simulink model "plotting_sim"  (R2014b)
settings: Solver=ode45  StartTime=0.0  StopTime=15  FixedStep=ts  RelTol=1e-3
values from neighbouring files (symbols this model uses):
  A = eval(As)    [plotting_script.m]
  B = eval(Bs)    [plotting_script.m]
  Cc = eye(5,6)    [plotting_script.m]
  Kr = (-inv(Cs*inv(Aa-Bb*K)*Bb))    [plotting_script.m]
undefined symbols (not defined in the file or in its folder): K, sigbuilder_block
settings Model: CovSFcnEnable=on  Creator=Jaby  LastModifiedBy=danielpihlquist
settings OptimizationCC: UseDivisionForNetSlopeComputation=off  SimCompilerOptimization=off
settings DebuggingCC: SolverPrmCheckMsg=none  FrameProcessingCompatibilityMsg=error
settings RTWCC: RTWCompilerOptimization=off

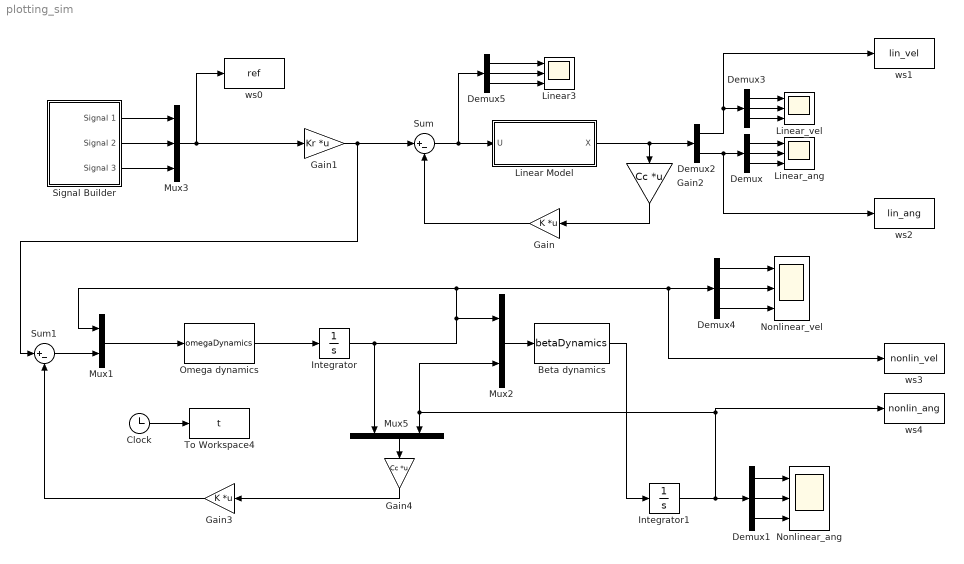
== system plotting_sim ==
  Beta dynamics : MATLABFcn  MATLABFcn=betaDynamics  Output1D=off
  Clock : Clock
  Demux{,1,3..5} (5 alike) : Demux  Outputs=3
  Demux2 : Demux  Outputs=2
  Gain : Gain  Gain=K  Multiplication=Matrix(K*u)
  Gain1 : Gain  Gain=Kr  Multiplication=Matrix(K*u)
  Gain2 : Gain  Gain=Cc  Multiplication=Matrix(K*u)
  Gain3 : Gain  Gain=K  Multiplication=Matrix(K*u)
  Gain4 : Gain  Gain=Cc  Multiplication=Matrix(K*u)
  Integrator : Integrator  InitialCondition=[0 0 0]'
  Integrator1 : Integrator  InitialCondition=[0 0 0]'
  "Linear Model " : Subsystem
  Linear3 : Scope  NumInputPorts=3
      settings: TimeRange=20  YMin=0.00274~-3.07e-14~8.3e-31  YMax=0.00278~-3.025e-14~8.43e-31  SaveName=ScopeData4
  Linear_ang : Scope  NumInputPorts=3
      settings: TimeRange=20  YMin=0.00274~-3.07e-14~8.3e-31  YMax=0.00278~-3.025e-14~8.43e-31
  Linear_vel : Scope  NumInputPorts=3
      settings: TimeRange=20  YMin=-0.5~-0.5~0  YMax=2.5~2.5~0.7000000000000001  SaveName=ScopeData2
  Mux1 : Mux  Inputs=2
  Mux2 : Mux  Inputs=2
  Mux3 : Mux  Inputs=3
  Mux5 : Mux  Inputs=2
  "Nonlinear_ang " : Scope  NumInputPorts=3
      settings: YMin=-5~-5~-5  YMax=5~5~5
  Nonlinear_vel : Scope  NumInputPorts=3
      settings: YMin=-5~-5~-5  YMax=5~5~5  SaveName=ScopeData3
  Omega dynamics : MATLABFcn  MATLABFcn=omegaDynamics  Output1D=off
  Signal Builder : Subsystem  Tag=STV Subsys  LoadFcn=sigbuilder_block('load');  StartFcn=sigbuilder_block('start');  StopFcn=sigbuilder_block('stop');  ClipboardFcn=sigbuilder_block('clipboard');  mask(Sigbuilder block){}
      mask help: Simulink:masks:SigbuilderBlock_MD
      mask init:
      | if ~strcmp(get_param(bdroot(gcbh),'SimulationStatus'),'stopped') tuvar = sigbuilder_block('maskInit'); end
      settings: CopyFcn=sigbuilder_block('copy');  DeleteFcn=sigbuilder_block('delete');  ModelCloseFcn=sigbuilder_block('modelClose');  PreSaveFcn=sigbuilder_block('preSave');  PauseFcn=sigbuilder_block('pause');  ContinueFcn=sigbuilder_block('continue');  NameChangeFcn=sigbuilder_block('namechange');  OpenFcn=sigbuilder_block('open',[437.6 199.2 550.4 400 ]);  CloseFcn=sigbuilder_block('close');
      mask Display: plot(0, 0, 100, 100,[2, 2, 32, 32, 2], [68, 8, 8, 68, 68],[32, 2], [38, 38], [32, 19, 2],[53, 60, 44], [32, 17, 17, 2],[16, 16, 31, 31]);txt = getActiveGroup(gcbh);text(2, 100, txt,'verticalAlignment', 'top');
  Sum : Sum  Inputs=|+-
  Sum1 : Sum  Inputs=|+-
  To Workspace4 : ToWorkspace  VariableName=t  SampleTime=-1
  ws0 : ToWorkspace  VariableName=ref  SampleTime=-1
  ws1 : ToWorkspace  VariableName=lin_vel  SampleTime=-1
  ws2 : ToWorkspace  VariableName=lin_ang  SampleTime=-1
  ws3 : ToWorkspace  VariableName=nonlin_vel  SampleTime=-1
  ws4 : ToWorkspace  VariableName=nonlin_ang  SampleTime=-1
  wires:
  Demux/1 -> Linear_ang/1
  Demux/2 -> Linear_ang/2
  Demux/3 -> Linear_ang/3
  Integrator/1 -> Demux4/1, ws3/1, Mux1/1, Mux2/1, Mux5/1
  Mux1/1 -> Omega dynamics/1
  Omega dynamics/1 -> Integrator/1
  Beta dynamics/1 -> Integrator1/1
  Demux1/2 -> "Nonlinear_ang "/2
  Demux1/3 -> "Nonlinear_ang "/3
  Demux1/1 -> "Nonlinear_ang "/1
  Gain/1 -> Sum/2
  Demux2/2 -> Demux/1, ws2/1
  Signal Builder/2(Signal 2) -> Mux3/2
  Signal Builder/1(Signal 1) -> Mux3/1
  Demux3/1 -> Linear_vel/1
  Demux3/2 -> Linear_vel/2
  Demux3/3 -> Linear_vel/3
  Signal Builder/3(Signal 3) -> Mux3/3
  "Linear Model "/1(X) -> Demux2/1, Gain2/1
  Gain1/1 -> Sum1/1, Sum/1
  Demux5/1 -> Linear3/1
  Demux5/2 -> Linear3/2
  Demux5/3 -> Linear3/3
  Sum/1 -> Demux5/1, "Linear Model "/1(U)
  Gain2/1 -> Gain/1
  Gain4/1 -> Gain3/1
  Gain3/1 -> Sum1/2
  Sum1/1 -> Mux1/2
  Mux5/1 -> Gain4/1
  Demux4/2 -> Nonlinear_vel/2
  Mux2/1 -> Beta dynamics/1
  Demux4/3 -> Nonlinear_vel/3
  Demux4/1 -> Nonlinear_vel/1
  Mux3/1 -> Gain1/1, ws0/1
  Demux2/1 -> Demux3/1, ws1/1
  Integrator1/1 -> Demux1/1, ws4/1, Mux5/2, Mux2/2
  Clock/1 -> To Workspace4/1

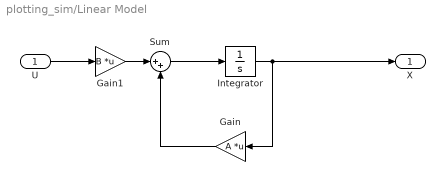
== system plotting_sim/Linear Model  ==
  U : Inport
  Gain : Gain  Gain=A  Multiplication=Matrix(K*u)
  Gain1 : Gain  Gain=B  Multiplication=Matrix(K*u)
  Integrator : Integrator
  Sum : Sum  Inputs=|++
  X : Outport
  wires:
  Integrator/1 -> X/1, Gain/1
  U/1 -> Gain1/1
  Gain1/1 -> Sum/1
  Sum/1 -> Integrator/1
  Gain/1 -> Sum/2

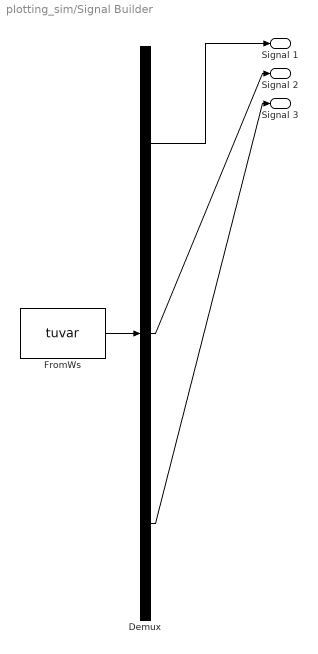
== system plotting_sim/Signal Builder ==
  Demux : Demux  Tag=STV Demux  Outputs=3
  FromWs : FromWorkspace  Tag=STV FromWs  VariableName=tuvar  SampleTime=0
      SigBuilderData=|
      | common.afterFinalStr = 'Extrapolate'
      | common.sampleTime = 0
      | dataSet.timeRange = [0 10]
      | dataSet.name = 'Group 1'
      | sbobj.Groups.Name = 'Group 1'
      | sbobj.Groups.Signals(1).Name = 'Signal 1'
      | sbobj.Groups.Signals(1).XData = [0 0.86 0.86 2.86 2.86 10]
      | sbobj.Groups.Signals(1).YData = [0 0 1 1 0 0]
      | sbobj.Groups.Signals(2).Name = 'Signal 2'
      | sbobj.Groups.Signals(2).XData = [0 3.94 3.94 10]
      | sbobj.Groups.Signals(2).YData = [0 0 1 1]
      | sbobj.Groups.Signals(3).Name = 'Signal 3'
      | sbobj.Groups.Signals(3).XData = [0 5.76 5.76 9.98 9.98 10]
      | sbobj.Groups.Signals(3).YData = [0 0 1 1 0 0]
  Signal 1 : Outport  Tag=STV Outport
  Signal 2 : Outport  Tag=STV Outport  Port=2
  Signal 3 : Outport  Tag=STV Outport  Port=3
  wires:
  Demux/1 -> Signal 1/1
  FromWs/1 -> Demux/1
  Demux/2 -> Signal 2/1
  Demux/3 -> Signal 3/1
